simulink model "BenchtopSkinpatch_SingleTone_HDL"  (R2016a)
settings: Solver=FixedStepDiscrete  SolverMode=SingleTasking  StartTime=0.0  StopTime=sim_time  RelTol=1e-3
undefined symbols (not defined in the file): bitrevorder, CFC_FFTlength, designMultirateFIR, Ts
libraries: dspsigops x8, simulink x4, commdigbbndpm3 x1, dsparch4 x1, dspxfrm3 x1, hdlsllib x1, dspmlti4 x1
settings Model: Creator=ckilfoyl  LastModifiedBy=Larson_Lab_Brown
settings DataIOCC: SaveOutput=off  SignalLogging=off  DSMLogging=off  SaveTime=off  LoggingToFile=on
settings OptimizationCC: BlockReduction=off  ConditionallyExecuteInputs=off  DefaultParameterBehavior=Inlined
settings DebuggingCC: AlgebraicLoopMsg=error  SingleTaskRateTransMsg=error
settings HardwareCC: ProdBitPerPointer=32  ProdLargestAtomicFloat=None  ProdIntDivRoundTo=Undefined  ProdEndianess=Unspecified  ProdWordSize=32  ProdHWDeviceType=ASIC/FPGA->ASIC/FPGA  ProdEqTarget=off

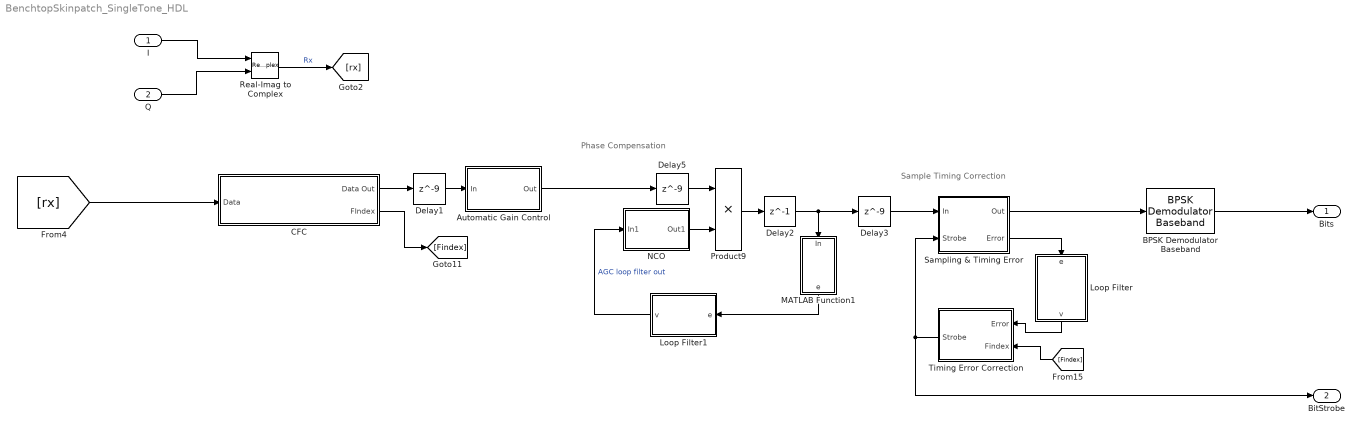
== system BenchtopSkinpatch_SingleTone_HDL ==
  note: Phase Compensation
  note: Sample Timing Correction
  I : Inport  OutDataTypeStr=fixdt(1,16,14)  PortDimensions=1  SampleTime=Ts
  Q : Inport  Port=2  OutDataTypeStr=fixdt(1,16,14)  PortDimensions=1  SampleTime=Ts
  Automatic Gain Control : Subsystem  mask{AGCLoopGain=1, AGCUpperLimit=1000, AGCRef=1}
      mask prompts: AGCLoopGain "Loop Gain"; AGCUpperLimit "Maximum Gain"; AGCRef "Desired Amplitude"
  BPSK Demodulator Baseband : commdigbbndpm3/BPSK Demodulator Baseband  DecType=Hard decision  VarSource=Dialog  Variance=1  Ph=0  outDtype=Inherit via internal rule  derotateFactorWordLen=16  derotateFactorDataTypeStr=Inherit: Same word length as input  derotateFactorLastDataTypeStr=Inherit: Same word length as input
  CFC : Subsystem
  Delay1 : Delay  DelayLength=9  InitialCondition=0
  Delay2 : Delay  DelayLength=1  InitialCondition=0
  Delay3 : Delay  DelayLength=9  InitialCondition=0
  Delay5 : Delay  DelayLength=9  InitialCondition=0
  Loop Filter : Subsystem  mask{BnTs=.1, zeta=2, N=12, Kp=0.5, K0=1}
      mask prompts: BnTs "Normalized Loop Bandwidth"; zeta "Damping Factor"; N "Number of Samples/Symbol"; Kp "Phase Detector Gain (Kp)"; K0 "DDS Gain (K0)"
      mask init:
      | % See C.57 to C.61 in Michael Rice's "Digital Communications 
      | % - A Discrete-Time Approach" for details
      | theta = BnTs/(zeta+0.25/zeta)/N;
      | d = 1 + 2*zeta*theta + theta*theta;
      | K1 = 4*zeta*theta/d;
      | K2 = 4*theta*theta/d;
      | K1 = K1/(Kp*K0);
      | K2 = K2/(Kp*K0);
      mask Display: disp('Loop Filter')
  Loop Filter1 : Subsystem  mask{BnTs=.1, zeta=2.5, N=12, Kp=2, K0=1}
      mask prompts: BnTs "Normalized Loop Bandwidth"; zeta "Damping Factor"; N "Number of Samples/Symbol"; Kp "Phase Detector Gain (Kp)"; K0 "DDS Gain (K0)"
      mask init: same as BenchtopSkinpatch_SingleTone_HDL/Loop Filter
      mask Display: disp('Loop Filter')
  MATLAB Function1 : MATLAB Function  TreatAsAtomicUnit=on
  NCO : Subsystem
  Product9 : Product  OutDataTypeStr=fixdt(1,16,14)  SaturateOnIntegerOverflow=on  RndMeth=Zero
  Real-Imag to Complex : RealImagToComplex
  Sampling & Timing Error : Subsystem
  Timing Error Correction : Subsystem
  Bits : Outport
  BitStrobe : Outport  Port=2
  wires:
  I/1 -> Real-Imag to Complex/1
  Q/1 -> Real-Imag to Complex/2
  Real-Imag to Complex/1 -> [rx]  "Rx"
  Sampling & Timing Error/1(Out) -> BPSK Demodulator Baseband/1
  BPSK Demodulator Baseband/1 -> Bits/1
  Delay5/1 -> Product9/1
  Product9/1 -> Delay2/1
  MATLAB Function1/1(e) -> Loop Filter1/1(e)
  NCO/1(Out1) -> Product9/2
  Loop Filter1/1(v) -> NCO/1(In1)  "AGC loop filter out"
  Sampling & Timing Error/2(Error) -> Loop Filter/1(e)
  Timing Error Correction/1(Strobe) -> BitStrobe/1, Sampling & Timing Error/2(Strobe)
  Loop Filter/1(v) -> Timing Error Correction/1(Error)
  Delay2/1 -> Delay3/1, MATLAB Function1/1(In)
  Automatic Gain Control/1(Out) -> Delay5/1
  CFC/2(FIndex) -> [Findex]
  [Findex] -> Timing Error Correction/2(Findex)
  [rx] -> CFC/1(Data)
  CFC/1(Data Out) -> Delay1/1
  Delay1/1 -> Automatic Gain Control/1(In)
  Delay3/1 -> Sampling & Timing Error/1(In)

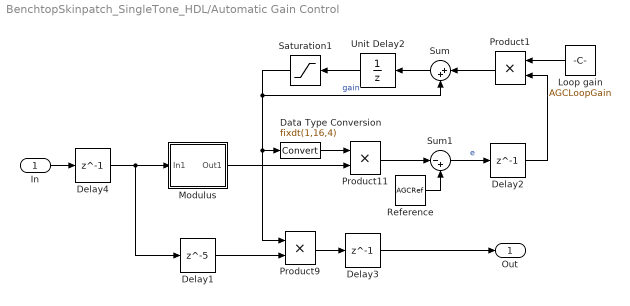
== system BenchtopSkinpatch_SingleTone_HDL/Automatic Gain Control ==
  In : Inport
  Data Type Conversion : DataTypeConversion  OutDataTypeStr=fixdt(1,16,4)  SaturateOnIntegerOverflow=on
  Delay1 : Delay  DelayLength=5  InitialCondition=0
  Delay2 : Delay  DelayLength=1  InitialCondition=0
  Delay3 : Delay  DelayLength=1  InitialCondition=0
  Delay4 : Delay  DelayLength=1  InitialCondition=0
  Loop gain : Constant  Value=AGCLoopGain  OutDataTypeStr=fixdt(1,16,10)  SampleTime=Ts
  Modulus : Subsystem
  Product1 : Product  OutDataTypeStr=fixdt(1,16,10)  RndMeth=Zero
  Product11 : Product  OutDataTypeStr=fixdt(1,16,10)  RndMeth=Zero
  Product9 : Product  OutDataTypeStr=fixdt(1,16,14)  SaturateOnIntegerOverflow=on  RndMeth=Zero
  Reference : Constant  Value=AGCRef  OutDataTypeStr=fixdt(1,16,10)  SampleTime=Ts
  Saturation1 : Saturate  UpperLimit=AGCUpperLimit  LowerLimit=1e-5
  Sum : Sum  Inputs=|++  OutDataTypeStr=fixdt(1,23,10)  SaturateOnIntegerOverflow=on
  Sum1 : Sum  Inputs=|-+  OutDataTypeStr=Inherit: Same as first input
  Unit Delay2 : UnitDelay  SampleTime=-1
  Out : Outport  PortDimensions=1
  wires:
  Saturation1/1 -> Sum/2, Product9/1, Data Type Conversion/1  "gain"
  Loop gain/1 -> Product1/1
  Product1/1 -> Sum/1
  Modulus/1(Out1) -> Product11/2
  Delay4/1 -> Modulus/1(In1), Delay1/1
  Unit Delay2/1 -> Saturation1/1
  Delay2/1 -> Product1/2
  Delay3/1 -> Out/1
  Delay1/1 -> Product9/2
  Product9/1 -> Delay3/1
  Sum1/1 -> Delay2/1  "e"
  Sum/1 -> Unit Delay2/1
  Reference/1 -> Sum1/2
  Data Type Conversion/1 -> Product11/1
  Product11/1 -> Sum1/1
  In/1 -> Delay4/1

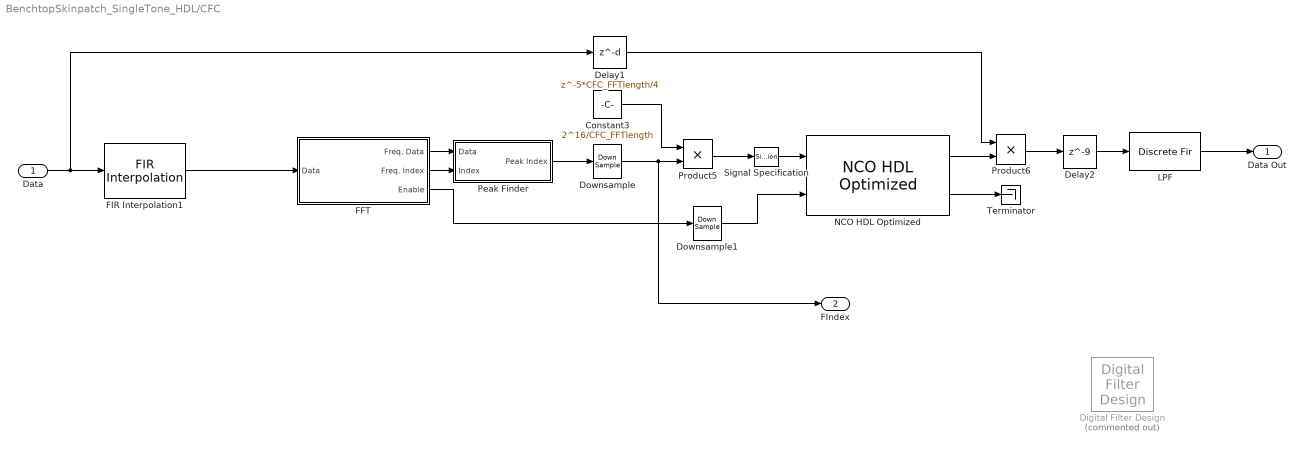
== system BenchtopSkinpatch_SingleTone_HDL/CFC ==
  Data : Inport
  Constant3 : Constant  Value=2^16/CFC_FFTlength  OutDataTypeStr=int16
  Delay1 : Delay  DelayLength=5*CFC_FFTlength/4  InitialCondition=0  SampleTime=Ts
  Delay2 : Delay  DelayLength=9  InitialCondition=0
  Digital Filter Design : dsparch4/Digital Filter Design  Commented=on  mwdsp_browser_bugfix_var=off
  Downsample : DownSample  RateOptions=Allow multirate processing
  Downsample1 : DownSample  RateOptions=Allow multirate processing
  FFT : Subsystem
  FIR Interpolation1 : dspmlti4/FIR Interpolation  FilterSource=Auto  h=designMultirateFIR(3,1)  L=2  FilterObject=FINTERP  framing=Allow multirate processing  outputBufInitCond=0  roundingMode=Floor  overflowMode=off  firstCoeffDataTypeStr=Inherit: Same word length as input  firstCoeffMin=[]  firstCoeffMax=[]  firstCoeffLastDataTypeStr=Inherit: Same word length as input  outputMin=[]  outputMax=[]
  LPF : DiscreteFir  Tag=BlockMethodSubSystem  Coefficients=[-0.0013779689989745409 -0.0083115975069562534 -0.0050263173761967784 -0.0063818336562817867 -0.0058948557787365562 -0.0046922766501128702 -0.0027829648788689795 -0.00060452121700571505 0.001354682158452473 0.0026429859496680448 0.002975579677085971 0.0023269581355887096 0.00094106296298738623 -0.00072602390997707526 -0.0021435474084144719 -0.002854240021640119 -0.0026231311352084598 -0.0015099889418793843 0.00013891499904289116 0.0017985773125025269 0.0029193273982120842 0.0031151247201403397 0.0022823313666537055 0.00065483000269016657 -0.0012676041813121884 -0.0028640160668193461 -0.003591926189322013 -0.0031664272960530552 -0.0016710738469885046 0.00045843776922720484 0.0025489682662245233 0.0039099645185178425 0.0040510996505595202 0.0028611304203498915 0.00066003098671916279 -0.0018843144503149305 -0.0039512905636197651 -0.0048333301131551418 -0.0041672792968443064 -0.0020855963811220973 0.0008087644552933781 0.0036064079536425463 0.0053786714743630226 0.0054831928019420566 0.0037799724375766372 0.00072165625528820745 -0.0027708035160954477 -0.0055668153146814772 -0.0066968208429582631 -0.0056832843839253475 -0.0027214522278970351 0.0013443997730585484 0.0052426739552877315 0.0076716824392495681 0.0077212813832632033 0.0052121794929347728 0.00078606233985197634 -0.0042371034953577651 -0.0082334585626777489 -0.0097934643854344691 -0.0082163538236654076 -0.003764259594220568 0.0023269072667433041 0.0081648171083775929 0.011790310135765179 0.011798548105624229 0.0078332200083936539 0.00083920861866352984 -0.0071641371165231975 -0.013610280415778999 -0.016163815072196629 -0.013532513859394973 -0.0059504274198176671 0.004660114909203943 0.015158518753173443 0.021993163643765579 0.022300705242665805 0.014889969255362949 0.00087174589780205476 -0.016319854836857897 -0.031574523927105309 -0.039282005313476927 -0.034791115089744487 -0.015742672646747145 0.017049733584603807 0.059476947428655141 0.10481298102062764 0.14508835683571572 0.17281963611626916 0.18270340855975087 0.17281963611626916 0.14508835683571572 0.10481298102062764 0.059476947428655141 0.017049733584603807 -0.015742672646747145 -0.034791115089744487 -0.039282005313476927 -0.031574523927105309 -0.016319854836857897 0.00087174589780205476 0.014889969255362949 0.022300705242665805 0.021993163643765579 0.015158518753173443 0.004660114909203943 -0.0059504274198176671 -0.013532513859394973 -0.016163815072196629 -0.013610280415778999 -0.0071641371165231975 0.00083920861866352984 0.0078332200083936539 0.011798548105624229 0.011790310135765179 0.0081648171083775929 0.0023269072667433041 -0.003764259594220568 -0.0082163538236654076 -0.0097934643854344691 -0.0082334585626777489 -0.0042371034953577651 0.00078606233985197634 0.0052121794929347728 0.0077212813832632033 0.0076716824392495681 0.0052426739552877315 0.0013443997730585484 -0.0027214522278970351 -0.0056832843839253475 -0.0066968208429582631 -0.0055668153146814772 -0.0027708035160954477 0.00072165625528820745 0.0037799724375766372 0.0054831928019420566 0.0053786714743630226 0.0036064079536425463 0.0008087644552933781 -0.0020855963811220973 -0.0041672792968443064 -0.0048333301131551418 -0.0039512905636197651 -0.0018843144503149305 0.00066003098671916279 0.0028611304203498915 0.0040510996505595202 0.0039099645185178425 0.0025489682662245233 0.00045843776922720484 -0.0016710738469885046 -0.0031664272960530552 -0.003591926189322013 -0.0028640160668193461 -0.0012676041813121884 0.00065483000269016657 0.0022823313666537055 0.0031151247201403397 0.0029193273982120842 0.0017985773125025269 0.00013891499904289116 -0.0015099889418793843 -0.0026231311352084598 -0.002854240021640119 -0.0021435474084144719 -0.00072602390997707526 0.00094106296298738623 0.0023269581355887096 0.002975579677085971 0.0026429859496680448 0.001354682158452473 -0.00060452121700571505 -0.0027829648788689795 -0.0046922766501128702 -0.0058948557787365562 -0.0063818336562817867 -0.0050263173761967784 -0.0083115975069562534 -0.0013779689989745409]  InputProcessing=Columns as channels (frame based)
  NCO HDL Optimized : dspsigops/NCO HDL Optimized  PhaseIncrementSource=Input port  PhaseIncrement=100  PhaseOffsetSource=Property  PhaseOffset=0  DitherSource=Property  NumDitherBits=4  PhaseQuantization=on  NumQuantizerAccumulatorBits=12  LUTCompress=off  ResetAction=off  ValidInputPort=on  Waveform=Complex exponential  PhasePort=off  AccumulatorWL=16  OutputDataType=Binary point scaling  OutputWL=16  OutputFL=14  SimulateUsing=Code generation
  "Peak Finder " : Subsystem
  Product5 : Product  OutDataTypeStr=fixdt(1,16,0)
  Product6 : Product  OutDataTypeStr=fixdt(1,16,14)
  Signal Specification : SignalSpecification  OutDataTypeStr=fixdt(1,16,0)  Dimensions=1
  Terminator : Terminator
  Data Out : Outport
  FIndex : Outport  Port=2
  wires:
  Constant3/1 -> Product5/1
  Data/1 -> FIR Interpolation1/1, Delay1/1
  NCO HDL Optimized/1 -> Product6/2
  Downsample1/1 -> NCO HDL Optimized/2
  FFT/3(Enable) -> Downsample1/1
  FFT/1(Freq. Data) -> "Peak Finder "/1(Data)
  FFT/2(Freq. Index) -> "Peak Finder "/2(Index)
  FIR Interpolation1/1 -> FFT/1(Data)
  Delay1/1 -> Product6/1
  Product6/1 -> Delay2/1
  LPF/1 -> Data Out/1
  "Peak Finder "/1("Peak Index ") -> Downsample/1
  NCO HDL Optimized/2 -> Terminator/1
  Downsample/1 -> Product5/2, FIndex/1
  Signal Specification/1 -> NCO HDL Optimized/1
  Product5/1 -> Signal Specification/1
  Delay2/1 -> LPF/1

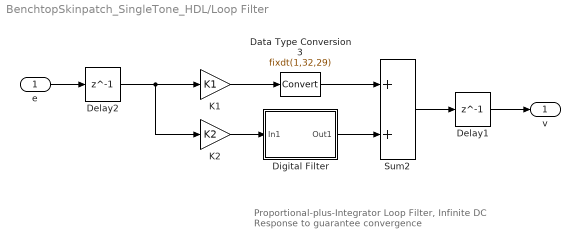
== system BenchtopSkinpatch_SingleTone_HDL/Loop Filter ==
  note: Proportional-plus-Integrator Loop Filter,
      | Infinite DC Response to guarantee convergence
  e : Inport
  Data Type Conversion3 : DataTypeConversion  OutDataTypeStr=fixdt(1,32,29)
  Delay1 : Delay  DelayLength=1  InitialCondition=0
  Delay2 : Delay  DelayLength=1  InitialCondition=0
  Digital Filter : Subsystem
  K1 : Gain  Gain=K1
  K2 : Gain  Gain=K2
  Sum2 : Sum  OutDataTypeStr=fixdt(1,22,19)  SaturateOnIntegerOverflow=on  InputSameDT=on
  v : Outport
  wires:
  Delay1/1 -> v/1
  Digital Filter/1(Out1) -> Sum2/2
  Sum2/1 -> Delay1/1
  K2/1 -> Digital Filter/1(In1)
  Data Type Conversion3/1 -> Sum2/1
  Delay2/1 -> K2/1, K1/1
  e/1 -> Delay2/1
  K1/1 -> Data Type Conversion3/1

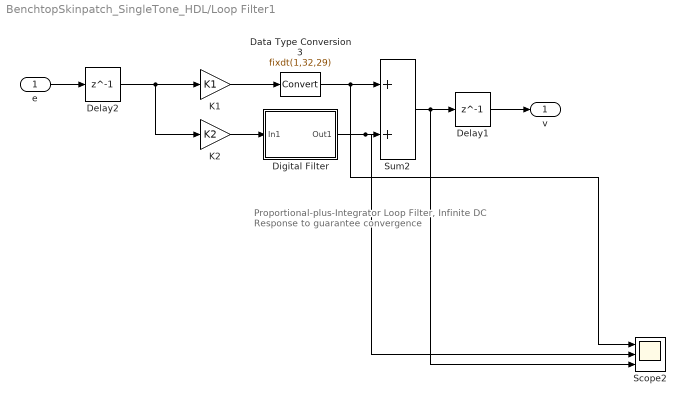
== system BenchtopSkinpatch_SingleTone_HDL/Loop Filter1 ==
  note: Proportional-plus-Integrator Loop Filter,
      | Infinite DC Response to guarantee convergence
  e : Inport
  Data Type Conversion3 : DataTypeConversion  OutDataTypeStr=fixdt(1,32,29)
  Delay1 : Delay  DelayLength=1  InitialCondition=0
  Delay2 : Delay  DelayLength=1  InitialCondition=0
  Digital Filter : Subsystem
  K1 : Gain  Gain=K1
  K2 : Gain  Gain=K2
  Scope2 : Scope  NumInputPorts=3
  Sum2 : Sum  OutDataTypeStr=fixdt(1,22,19)  SaturateOnIntegerOverflow=on  InputSameDT=on
  v : Outport
  wires:
  Delay1/1 -> v/1
  Digital Filter/1(Out1) -> Scope2/2, Sum2/2
  Sum2/1 -> Scope2/3, Delay1/1
  K2/1 -> Digital Filter/1(In1)
  Data Type Conversion3/1 -> Scope2/1, Sum2/1
  Delay2/1 -> K2/1, K1/1
  e/1 -> Delay2/1
  K1/1 -> Data Type Conversion3/1

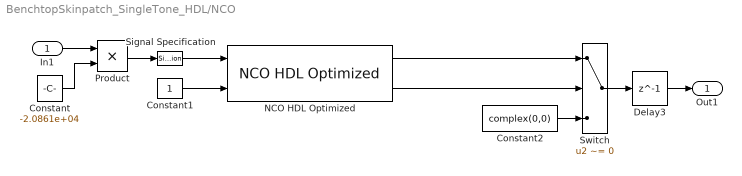
== system BenchtopSkinpatch_SingleTone_HDL/NCO ==
  In1 : Inport
  Constant : Constant  Value=-2.0861e+04  OutDataTypeStr=int16  SampleTime=Ts
  Constant1 : Constant  OutDataTypeStr=boolean  SampleTime=Ts
  Constant2 : Constant  Value=complex(0,0)  OutDataTypeStr=fixdt(1,10,8)  SampleTime=Ts
  Delay3 : Delay  DelayLength=1  InitialCondition=0
  NCO HDL Optimized : dspsigops/NCO HDL Optimized  PhaseIncrementSource=Input port  PhaseIncrement=100  PhaseOffsetSource=Property  PhaseOffset=0  DitherSource=None  NumDitherBits=1  PhaseQuantization=on  NumQuantizerAccumulatorBits=16  LUTCompress=on  ResetAction=off  ValidInputPort=on  Waveform=Complex exponential  PhasePort=off  AccumulatorWL=17  OutputDataType=Binary point scaling  OutputWL=10  OutputFL=8  SimulateUsing=Code generation
  Product : Product  OutDataTypeStr=int16
  Signal Specification : SignalSpecification  Dimensions=1
  Switch : Switch  Criteria=u2 ~= 0
  Out1 : Outport
  wires:
  Delay3/1 -> Out1/1
  Constant2/1 -> Switch/3
  NCO HDL Optimized/2 -> Switch/2
  Constant1/1 -> NCO HDL Optimized/2
  NCO HDL Optimized/1 -> Switch/1
  Signal Specification/1 -> NCO HDL Optimized/1
  Switch/1 -> Delay3/1
  Product/1 -> Signal Specification/1
  Constant/1 -> Product/2
  In1/1 -> Product/1

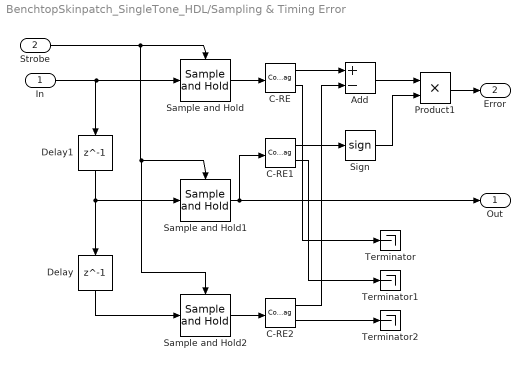
== system BenchtopSkinpatch_SingleTone_HDL/Sampling & Timing Error ==
  In : Inport
  Strobe : Inport  Port=2
  Add : Sum  Inputs=+-
  C-RE : ComplexToRealImag
  C-RE1 : ComplexToRealImag
  C-RE2 : ComplexToRealImag
  Delay : Delay  DelayLength=1  InitialCondition=0
  Delay1 : Delay  DelayLength=1  InitialCondition=0
  Product1 : Product
  Sample and Hold : dspsigops/Sample and Hold  trig=Rising edge  initCond=0  latchinput=off
  Sample and Hold1 : dspsigops/Sample and Hold  trig=Rising edge  initCond=0  latchinput=off
  Sample and Hold2 : dspsigops/Sample and Hold  trig=Rising edge  initCond=0  latchinput=off
  Sign : Signum
  Terminator : Terminator
  Terminator1 : Terminator
  Terminator2 : Terminator
  Out : Outport
  Error : Outport  Port=2
  wires:
  Delay1/1 -> Sample and Hold1/1, Delay/1
  Delay/1 -> Sample and Hold2/1
  Strobe/1 -> Sample and Hold2/Trigger, Sample and Hold1/Trigger, Sample and Hold/Trigger
  Sign/1 -> Product1/2
  Add/1 -> Product1/1
  Sample and Hold1/1 -> Out/1, C-RE1/1
  In/1 -> Delay1/1, Sample and Hold/1
  Product1/1 -> Error/1
  Sample and Hold/1 -> C-RE/1
  C-RE/1 -> Add/1
  C-RE2/1 -> Add/2
  Sample and Hold2/1 -> C-RE2/1
  C-RE1/1 -> Sign/1
  C-RE2/2 -> Terminator2/1
  C-RE1/2 -> Terminator1/1
  C-RE/2 -> Terminator/1

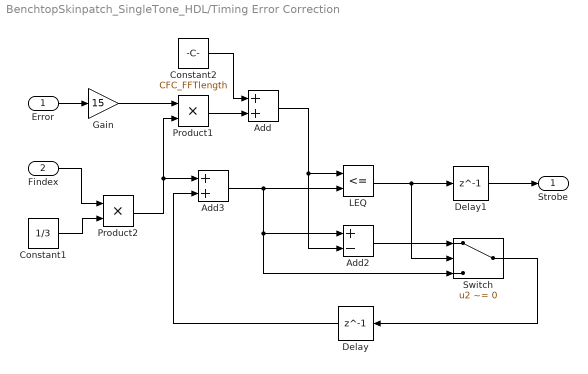
== system BenchtopSkinpatch_SingleTone_HDL/Timing Error Correction ==
  Error : Inport
  Findex : Inport  Port=2
  Add : Sum  OutDataTypeStr=int16
  Add2 : Sum  Inputs=+-
  Add3 : Sum  OutDataTypeStr=int16
  Constant1 : Constant  Value=1/3  OutDataTypeStr=fixdt(1,16,15)  SampleTime=-1
  Constant2 : Constant  Value=CFC_FFTlength  OutDataTypeStr=int16  SampleTime=-1
  Delay : Delay  DelayLength=1  InitialCondition=0
  Delay1 : Delay  DelayLength=1  InitialCondition=0
  Gain : Gain  Gain=15
  LEQ : RelationalOperator  Operator=<=  OutDataTypeStr=boolean
  Product1 : Product  OutDataTypeStr=int16
  Product2 : Product  OutDataTypeStr=int16
  Switch : Switch  Criteria=u2 ~= 0
  Strobe : Outport
  wires:
  Add/1 -> Add2/2, LEQ/1
  Add2/1 -> Switch/1
  Error/1 -> Gain/1
  Constant2/1 -> Add/1
  Add3/1 -> Switch/3, Add2/1, LEQ/2
  Switch/1 -> Delay/1
  Product1/1 -> Add/2
  LEQ/1 -> Delay1/1, Switch/2
  Delay/1 -> Add3/2
  Delay1/1 -> Strobe/1
  Gain/1 -> Product1/1
  Findex/1 -> Product2/1
  Constant1/1 -> Product2/2
  Product2/1 -> Product1/2, Add3/1

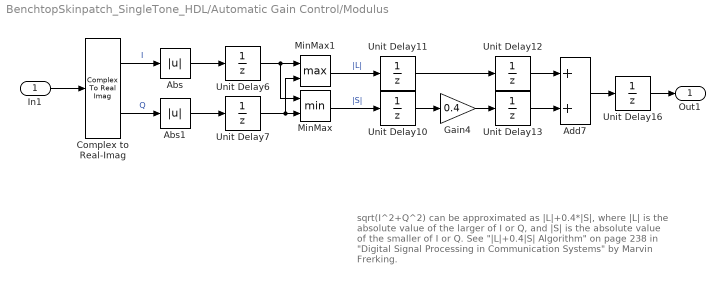
== system BenchtopSkinpatch_SingleTone_HDL/Automatic Gain Control/Modulus ==
  note: sqrt(I^2+Q^2) can be approximated as |L|+0.4*|S|,
      | where |L| is the absolute value of the larger of I or Q,
      | and |S| is the absolute value of the smaller of I or Q.
      |
      | See "|L|+0.4|S| Algorithm" on page 238 in "Digital Signal
      | Processing in Communication Systems" by Marvin Frerking.
  In1 : Inport
  Abs : Abs
  Abs1 : Abs
  Add7 : Sum
  Complex to Real-Imag : ComplexToRealImag
  Gain4 : Gain  Gain=0.4  OutDataTypeStr=fixdt(1,16,15)
  MinMax : MinMax  Inputs=2
  MinMax1 : MinMax  Function=max  Inputs=2
  Unit Delay{6..7,10..13,16} (7 alike) : UnitDelay  SampleTime=-1
  Out1 : Outport
  wires:
  In1/1 -> Complex to Real-Imag/1
  Unit Delay7/1 -> MinMax/2, MinMax1/2
  Unit Delay6/1 -> MinMax1/1, MinMax/1
  MinMax/1 -> Unit Delay10/1  "|S|"
  Gain4/1 -> Unit Delay13/1
  Unit Delay13/1 -> Add7/2
  MinMax1/1 -> Unit Delay11/1  "|L|"
  Complex to Real-Imag/2 -> Abs1/1  "Q"
  Complex to Real-Imag/1 -> Abs/1  "I"
  Abs/1 -> Unit Delay6/1
  Add7/1 -> Unit Delay16/1
  Abs1/1 -> Unit Delay7/1
  Unit Delay12/1 -> Add7/1
  Unit Delay10/1 -> Gain4/1
  Unit Delay16/1 -> Out1/1
  Unit Delay11/1 -> Unit Delay12/1

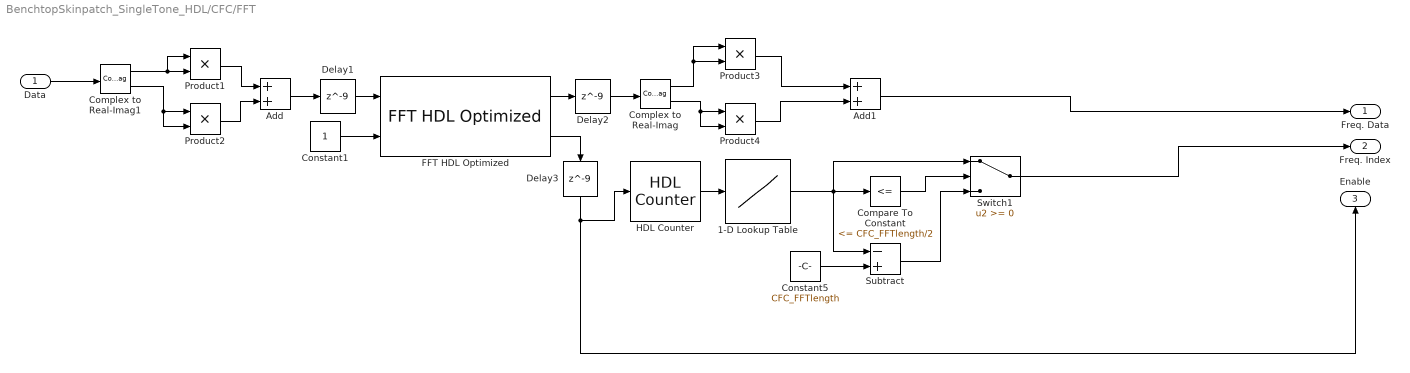
== system BenchtopSkinpatch_SingleTone_HDL/CFC/FFT ==
  Data : Inport
  1-D Lookup Table : Lookup_n-D  NumberOfTableDimensions=1  BreakpointsForDimension1=[0:(CFC_FFTlength - 1)]  BreakpointsForDimension1FirstPoint=10  BreakpointsForDimension2FirstPoint=10  BreakpointsForDimension1Spacing=12  BreakpointsForDimension2Spacing=12  IndexSearchMethod=Evenly spaced points  Table=bitrevorder(0:(CFC_FFTlength - 1))  InterpMethod=Flat  DiagnosticForOutOfRangeInput=Error  InternalRulePriority=Speed  OutDataTypeStr=int16  RndMeth=Simplest  InputSameDT=on
  Add : Sum  OutDataTypeStr=fixdt(1,16,14)
  Add1 : Sum  OutDataTypeStr=fixdt(1,16,14)
  Compare To Constant : simulink/Logic and Bit Operations/Compare To Constant  relop=<=  const=CFC_FFTlength/2  OutDataTypeStr=boolean
  Complex to Real-Imag : ComplexToRealImag
  Complex to Real-Imag1 : ComplexToRealImag
  Constant1 : Constant  OutDataTypeStr=boolean
  Constant5 : Constant  Value=CFC_FFTlength  OutDataTypeStr=int16
  Delay1 : Delay  DelayLength=9  InitialCondition=0
  Delay2 : Delay  DelayLength=9  InitialCondition=0
  Delay3 : Delay  DelayLength=9  InitialCondition=0
  FFT HDL Optimized : dspxfrm3/FFT HDL Optimized  Architecture=Streaming Radix 2^2  ComplexMultiplication=Use 3 multipliers and 5 adders  BitReversedOutput=on  Normalize=off  FFTLength=CFC_FFTlength  RoundingMethod=Floor  ResetInputPort=off  StartOutputPort=off  EndOutputPort=off  SimulateUsing=Code generation
  HDL Counter : hdlsllib/HDL Operations/HDL Counter  CountType=Free running  CountInit=0  CountStep=1  CountMax=25  CountFromType=Initial value  CountFrom=0  CountResetPort=off  CountLoadPort=off  CountEnbPort=on  CountDirPort=off  CountDataType=Unsigned  CountWordLen=log2(CFC_FFTlength)  CountFracLen=0  CountSampTime=1
  Product{1..4} (4 alike) : Product  OutDataTypeStr=fixdt(1,16,14)
  Subtract : Sum  Inputs=-+  OutDataTypeStr=int16
  Switch1 : Switch
  Freq. Data : Outport
  Freq. Index : Outport  Port=2
  Enable : Outport  Port=3
  wires:
  Product1/1 -> Add/1
  Product2/1 -> Add/2
  Constant1/1 -> FFT HDL Optimized/2
  Add1/1 -> Freq. Data/1
  Switch1/1 -> Freq. Index/1
  Product4/1 -> Add1/2
  Product3/1 -> Add1/1
  FFT HDL Optimized/1 -> Delay2/1
  Complex to Real-Imag/1 -> Product3/2, Product3/1
  Complex to Real-Imag/2 -> Product4/2, Product4/1
  Constant5/1 -> Subtract/2
  Add/1 -> Delay1/1
  FFT HDL Optimized/2 -> Delay3/1
  Compare To Constant/1 -> Switch1/2
  Subtract/1 -> Switch1/3
  Data/1 -> Complex to Real-Imag1/1
  Complex to Real-Imag1/1 -> Product1/1, Product1/2
  HDL Counter/1 -> 1-D Lookup Table/1
  Complex to Real-Imag1/2 -> Product2/2, Product2/1
  1-D Lookup Table/1 -> Subtract/1, Compare To Constant/1, Switch1/1
  Delay1/1 -> FFT HDL Optimized/1
  Delay2/1 -> Complex to Real-Imag/1
  Delay3/1 -> HDL Counter/1, Enable/1

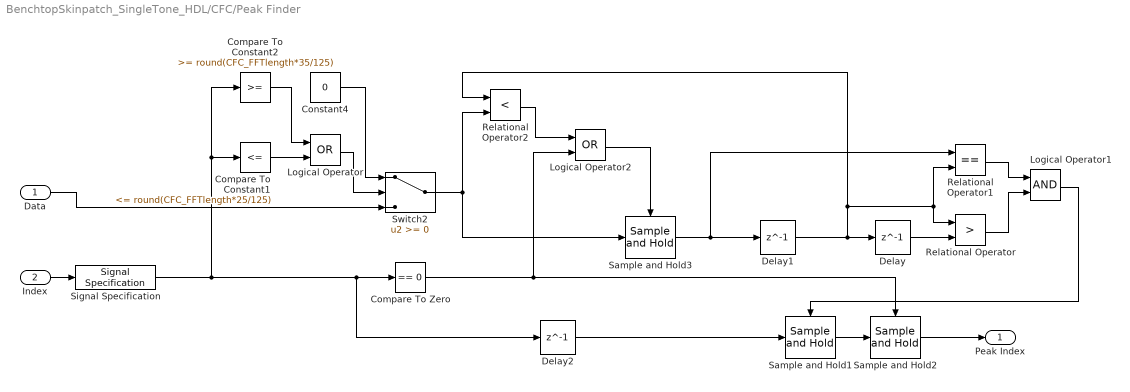
== system BenchtopSkinpatch_SingleTone_HDL/CFC/Peak Finder  ==
  Data : Inport
  Index : Inport  Port=2
  Compare To Constant1 : simulink/Logic and Bit Operations/Compare To Constant  relop=<=  const=round(CFC_FFTlength*25/125)  OutDataTypeStr=boolean
  Compare To Constant2 : simulink/Logic and Bit Operations/Compare To Constant  relop=>=  const=round(CFC_FFTlength*35/125)  OutDataTypeStr=boolean
  Compare To Zero : simulink/Logic and Bit Operations/Compare To Zero  relop===  OutDataTypeStr=boolean
  Constant4 : Constant  Value=0  OutDataTypeStr=fixdt(1,16,14)
  Delay : Delay  DelayLength=1  InitialCondition=0
  Delay1 : Delay  DelayLength=1  InitialCondition=0
  Delay2 : Delay  DelayLength=1  InitialCondition=0
  Logical Operator : Logic  Operator=OR  AllPortsSameDT=off  OutDataTypeStr=boolean
  Logical Operator1 : Logic  AllPortsSameDT=off  OutDataTypeStr=boolean
  Logical Operator2 : Logic  Operator=OR  AllPortsSameDT=off  OutDataTypeStr=boolean
  Relational Operator : RelationalOperator  Operator=>  OutDataTypeStr=boolean
  Relational Operator1 : RelationalOperator  Operator===  OutDataTypeStr=boolean
  Relational Operator2 : RelationalOperator  Operator=<  OutDataTypeStr=boolean
  Sample and Hold1 : dspsigops/Sample and Hold  trig=Rising edge  initCond=0  latchinput=off
  Sample and Hold2 : dspsigops/Sample and Hold  trig=Rising edge  initCond=0  latchinput=off
  Sample and Hold3 : dspsigops/Sample and Hold  trig=Rising edge  initCond=0  latchinput=off
  Signal Specification : SignalSpecification  OutDataTypeStr=int16  Dimensions=1
  Switch2 : Switch  OutDataTypeStr=fixdt(1,16,14)
  "Peak Index " : Outport
  wires:
  Data/1 -> Switch2/3
  Delay/1 -> Relational Operator/2
  Sample and Hold1/1 -> Sample and Hold2/1
  Switch2/1 -> Relational Operator2/2, Sample and Hold3/1
  Compare To Zero/1 -> Logical Operator2/2, Sample and Hold2/Trigger
  Compare To Constant2/1 -> Logical Operator/1
  Logical Operator/1 -> Switch2/2
  Constant4/1 -> Switch2/1
  Sample and Hold2/1 -> "Peak Index "/1
  Compare To Constant1/1 -> Logical Operator/2
  Index/1 -> Signal Specification/1
  Sample and Hold3/1 -> Relational Operator1/1, Delay1/1
  Signal Specification/1 -> Delay2/1, Compare To Zero/1, Compare To Constant2/1, Compare To Constant1/1
  Relational Operator1/1 -> Logical Operator1/1
  Relational Operator/1 -> Logical Operator1/2
  Logical Operator1/1 -> Sample and Hold1/Trigger
  Delay1/1 -> Relational Operator2/1, Relational Operator1/2, Relational Operator/1, Delay/1
  Delay2/1 -> Sample and Hold1/1
  Logical Operator2/1 -> Sample and Hold3/Trigger
  Relational Operator2/1 -> Logical Operator2/1

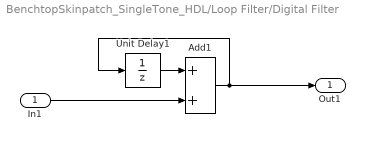
== system BenchtopSkinpatch_SingleTone_HDL/Loop Filter/Digital Filter ==
  In1 : Inport
  Add1 : Sum  OutDataTypeStr=fixdt(1,32,29)
  Unit Delay1 : UnitDelay  SampleTime=-1
  Out1 : Outport
  wires:
  Unit Delay1/1 -> Add1/1
  Add1/1 -> Out1/1, Unit Delay1/1
  In1/1 -> Add1/2

== system BenchtopSkinpatch_SingleTone_HDL/Loop Filter1/Digital Filter ==
  In1 : Inport
  Add1 : Sum  OutDataTypeStr=fixdt(1,32,29)
  Unit Delay1 : UnitDelay  SampleTime=-1
  Out1 : Outport
  wires:
  Unit Delay1/1 -> Add1/1
  Add1/1 -> Out1/1, Unit Delay1/1
  In1/1 -> Add1/2

== matlab function BenchtopSkinpatch_SingleTone_HDL/MATLAB Function1 ==
  data: In input; e output
function e  = PED(In)
% Input:
%   In - Input samples, oversampled by two
% Output:
%   e - Phase error
% PED implements 
% e = sign(imag(In)).*imag(In) - sign(real(In)).*real(In);

%#codegen

OP1 = real(In);
OP2 = imag(In);

Real = OP1;
Imag = OP2;

if(bitget(Real,16)==true)%real is negative
    OP1 = fi(-Imag,1,16,14);
end
if(bitget(Real,16)==false)%real is positive
    OP1 = fi(Imag,1,16,14);
end

e = fi(OP1,1,16,14);

% OP1 = real(In);
% OP2 = imag(In);
% 
% Real = OP1;
% Imag = OP2;
% OP3 = OP1;
% 
% if (bitget(Real,16)==false)%real part positive
%     OP1 = fi((1-Real),1,16,14);
%     OP2 = fi(Imag,1,16,14);
% end
% if (bitget(Real,16)==true)%real part negative
%     OP1 = fi(-(1+Real),1,16,14);
%     OP2 = fi(-Imag,1,16,14);
% end
% 
% if(bitget(Imag,16)==false)%imag part positive
%     OP3 = fi((OP2 + OP1)/2,1,16,14);
% end
% if(bitget(Imag,16)==true)%imag part negative
%     OP3 = fi((OP2 - OP1)/2,1,16,14);
% end
% 
% e= fi(OP3,1,16,14);
